simulink model "vector_model_submit_ver"  (R2023b)
settings: Solver=ode45  StartTime=0  StopTime=1  MaxStep=T_s  RelTol=1e-3  AbsTol=1e-3  EnableMultiTasking=on
values from neighbouring files (symbols this model uses):
  alpha_c = 2*pi*300    (= 1884.95559215)    [init_vector_submit_ver.m]
  alpha_s = 2*pi*20    (= 125.663706144)    [init_vector_submit_ver.m]
  J = 0.015    [init_vector_submit_ver.m]
  L_M = 0.224    [init_vector_submit_ver.m]
  L_sigma = 0.021    [init_vector_submit_ver.m]
  n_p = 2    [init_vector_submit_ver.m]
  psi_R_ref = 0.9    [init_vector_submit_ver.m]
  R_R = 2.1    [init_vector_submit_ver.m]
  T_L = 14.63    [init_vector_submit_ver.m]
  T_s = 125e-6    (= 0.000125)    [init_vector_submit_ver.m]
  tau_M_max = 20    [init_vector_submit_ver.m]
libraries: simulink x2
settings Model: Creator=mhinkkan  LastModifiedBy=Antti Jormanainen
settings SolverCC: AutoScaleAbsTol=off  AlgebraicLoopSolver=TrustRegion
settings DataIOCC: SaveFormat=Array  SignalLoggingSaveFormat=ModelDataLogs  SaveOutput=off  SignalLogging=off  DSMLogging=off  SaveTime=off  ReturnWorkspaceOutputs=off
settings OptimizationCC: BlockReduction=off  BooleanDataType=off  DefaultParameterBehavior=Inlined  OptimizeBlockIOStorage=off  BufferReuse=off  ReuseModelBlockBuffer=off  GlobalBufferReuse=off  ExpressionFolding=off  ExpressionDepthLimit=2147483647  LocalBlockOutputs=off  InitFltsAndDblsToZero=on  LifeSpan=inf
settings DebuggingCC: SaveWithParameterizedLinksMsg=none  UnderspecifiedInitializationDetection=Classic  MergeDetectMultiDrivingBlocksExec=none  SignalResolutionControl=TryResolveAllWithWarning  MultiTaskDSMMsg=warning  MultiTaskCondExecSysMsg=none  FcnCallInpInsideContextMsg=warning  UnconnectedInputMsg=warning  UnconnectedOutputMsg=warning  UnconnectedLineMsg=warning  StateNameClashWarn=warning  SFUnexpectedBacktrackingDiag=warning  SFNoUnconditionalDefaultTransitionDiag=warning  ArithmeticOperatorsInVariantConditions=warning
settings HardwareCC: ProdBitPerPointer=32  ProdBitPerSizeT=32  ProdBitPerPtrDiffT=32  ProdLargestAtomicFloat=None  ProdIntDivRoundTo=Undefined  ProdEndianess=Unspecified  ProdWordSize=32  ProdHWDeviceType=32-bit Generic  TargetUnknown=on
settings ModelReferenceCC: EnableRefExpFcnMdlSchedulingChecks=on  PropagateSignalLabelsOutOfModel=off
settings SFSimCC: SimUseLocalCustomCode=off  CustomCodeUndefinedFunction=UseInterfaceOnly
settings RTWCC: RTWUseLocalCustomCode=off
settings CodeAppCC: StateflowObjectComments=on
settings GRTTargetCC: TargetFcnLib=ansi_tfl_tmw.mat  TargetLangStandard=C89/C90 (ANSI)  CombineOutputUpdateFcns=off  GRTInterface=on
settings ConfigComp: CovMetricSettings=dw  CovSaveCumulativeToWorkspaceVar=on  CovSaveSingleToWorkspaceVar=on  CovExternalEMLEnable=off

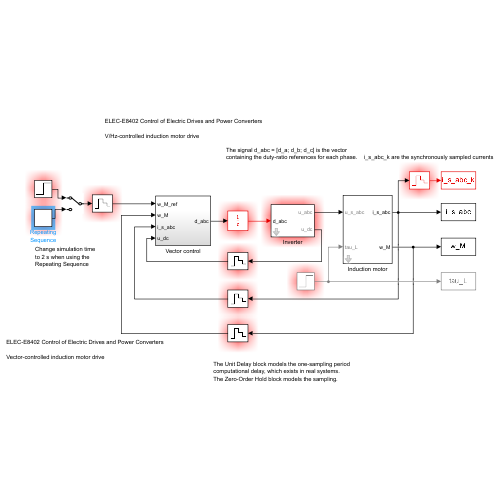
[thumbnail: Simulink's stored preview of the top-level diagram]
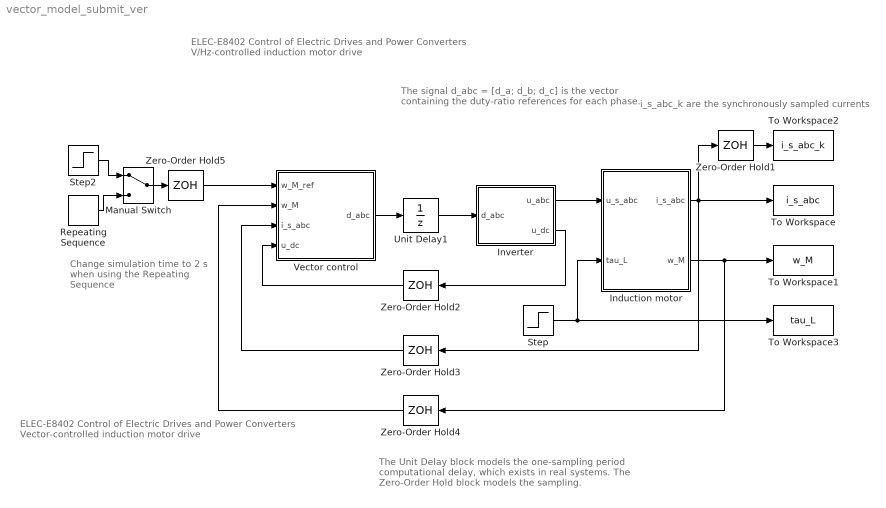
== system vector_model_submit_ver ==
  note: i_s_abc_k are the synchronously sampled currents
  note: The signal d_abc = [d_a; d_b; d_c] is the vector
      | containing the duty-ratio references for each phase.
  note: ELEC-E8402 Control of Electric Drives and Power Converters
      |
      | V/Hz-controlled induction motor drive
  note: The Unit Delay block models the one-sampling period
      | computational delay, which exists in real systems.
      | The Zero-Order Hold block models the sampling.
  note: Change simulation time
      | to 2 s when using the
      | Repeating Sequence
  note: ELEC-E8402 Control of Electric Drives and Power Converters
      |
      | Vector-controlled induction motor drive
  Induction motor : Subsystem  mask{R_s=3.7, R_R=2.1, L_sigma=0.021, L_M=0.224, n_p=2, J=0.015}
      mask prompts: R_s "Stator resistance R_s (ohm)"; R_R "Rotor resistance R_R (ohm)"; L_sigma "Leakage inductance L_sigma (H)"; L_M "Magnetizing inductance L_M (H)"; n_p "Number of pole pairs n_p"; J "Total inertia J (kgm^2)"
      mask help: Inverse-Gamma model
  Inverter : Subsystem  mask{T_s=T_s, u_dc=540}
      mask prompts: T_s "Sampling period T_s (s)"; u_dc "DC-link voltage u_dc (V)"
      mask help: The switching period is 2*Ts and the switching frequency is 1/(2*Ts).
  Manual Switch : ManualSwitch
  Repeating Sequence : simulink/Sources/Repeating Sequence  rep_seq_t=[0 .2 .8 1.2 1.8 2]  rep_seq_y=2*pi*30/n_p*[0 1 1 -1 -1 0]
  Step : Step  Time=.6  After=T_L  SampleTime=0
  Step2 : Step  Time=0.3  After=2*pi*40/n_p  SampleTime=T_s
  To Workspace : ToWorkspace  VariableName=i_s_abc  SaveFormat=Timeseries  SampleTime=-1
  To Workspace1 : ToWorkspace  VariableName=w_M  SaveFormat=Timeseries  SampleTime=-1
  To Workspace2 : ToWorkspace  VariableName=i_s_abc_k  SaveFormat=Timeseries  SampleTime=-1
  To Workspace3 : ToWorkspace  VariableName=tau_L  SaveFormat=Timeseries  SampleTime=-1
  Unit Delay1 : UnitDelay  SampleTime=T_s  HasFrameUpgradeWarning=on
  Vector control : Subsystem
  Zero-Order Hold{1..5} (5 alike) : ZeroOrderHold  SampleTime=T_s
  wires:
  Step/1 -> Induction motor/2(tau_L), To Workspace3/1
  Inverter/1(u_abc) -> Induction motor/1(u_s_abc)
  Induction motor/1(i_s_abc) -> Zero-Order Hold3/1, Zero-Order Hold1/1, To Workspace/1
  Induction motor/2(w_M) -> Zero-Order Hold4/1, To Workspace1/1
  Zero-Order Hold1/1 -> To Workspace2/1
  Manual Switch/1 -> Zero-Order Hold5/1
  Zero-Order Hold2/1 -> Vector control/4(u_dc)
  Repeating Sequence/1 -> Manual Switch/2
  Zero-Order Hold5/1 -> Vector control/1(w_M_ref)
  Step2/1 -> Manual Switch/1
  Vector control/1(d_abc) -> Unit Delay1/1
  Zero-Order Hold3/1 -> Vector control/3(i_s_abc)
  Zero-Order Hold4/1 -> Vector control/2(w_M)
  Unit Delay1/1 -> Inverter/1(d_abc)
  Inverter/2(u_dc) -> Zero-Order Hold2/1

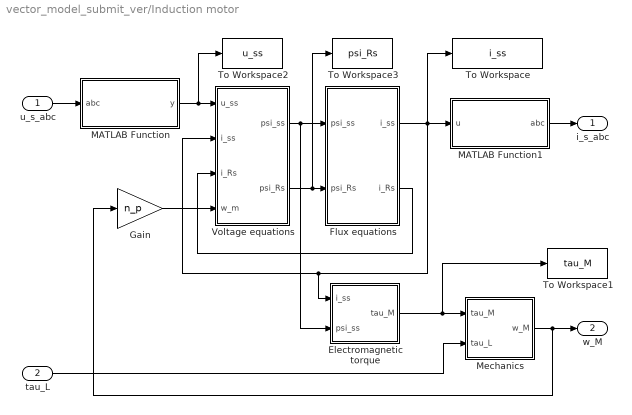
== system vector_model_submit_ver/Induction motor ==
  u_s_abc : Inport
  tau_L : Inport  Port=2
  Electromagnetic torque : Subsystem
  Flux equations : Subsystem
  Gain : Gain  Gain=n_p  SaturateOnIntegerOverflow=on  OutDataTypeStr=Inherit: Same as input  ParamDataTypeStr=Inherit: Same as input
  MATLAB Function : MATLAB Function  TreatAsAtomicUnit=on
  MATLAB Function1 : MATLAB Function  TreatAsAtomicUnit=on
  Mechanics : Subsystem
  To Workspace : ToWorkspace  VariableName=i_ss  SaveFormat=Timeseries  SampleTime=-1
  To Workspace1 : ToWorkspace  VariableName=tau_M  SaveFormat=Timeseries  SampleTime=-1
  To Workspace2 : ToWorkspace  VariableName=u_ss  SaveFormat=Timeseries  SampleTime=-1
  To Workspace3 : ToWorkspace  VariableName=psi_Rs  SaveFormat=Timeseries  SampleTime=-1
  Voltage equations : Subsystem
  i_s_abc : Outport
  w_M : Outport  Port=2
  wires:
  tau_L/1 -> Mechanics/2(tau_L)
  Mechanics/1(w_M) -> w_M/1, Gain/1
  Flux equations/1(i_ss) -> To Workspace/1, MATLAB Function1/1(u), Voltage equations/2(i_ss), Electromagnetic torque/1(i_ss)
  u_s_abc/1 -> MATLAB Function/1(abc)
  Voltage equations/2(psi_Rs) -> To Workspace3/1, Flux equations/2(psi_Rs)
  Voltage equations/1(psi_ss) -> Electromagnetic torque/2(psi_ss), Flux equations/1(psi_ss)
  Flux equations/2(i_Rs) -> Voltage equations/3(i_Rs)
  Electromagnetic torque/1(tau_M) -> To Workspace1/1, Mechanics/1(tau_M)
  MATLAB Function/1(y) -> To Workspace2/1, Voltage equations/1(u_ss)
  MATLAB Function1/1(abc) -> i_s_abc/1
  Gain/1 -> Voltage equations/4(w_m)

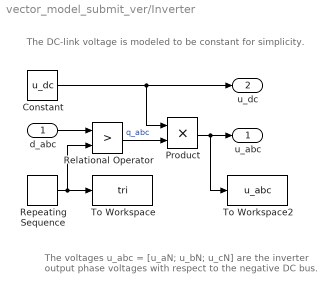
== system vector_model_submit_ver/Inverter ==
  note: The voltages u_abc = [u_aN; u_bN; u_cN] are the inverter
      | output phase voltages with respect to the negative DC bus.
  note: The DC-link voltage is modeled to be constant for simplicity.
  d_abc : Inport
  Constant : Constant  Value=u_dc  SampleTime=0
  Product : Product
  Relational Operator : RelationalOperator  Operator=>  OutDataTypeStr=boolean  InputSameDT=off
  Repeating Sequence : simulink/Sources/Repeating Sequence  rep_seq_t=[0 1 2]*T_s  rep_seq_y=[1 0 1]
  To Workspace : ToWorkspace  VariableName=tri  SaveFormat=Timeseries  SampleTime=-1
  To Workspace2 : ToWorkspace  VariableName=u_abc  SaveFormat=Timeseries  SampleTime=-1
  u_abc : Outport
  u_dc : Outport  Port=2
  wires:
  Repeating Sequence/1 -> Relational Operator/2, To Workspace/1
  d_abc/1 -> Relational Operator/1
  Relational Operator/1 -> Product/2  "q_abc"
  Constant/1 -> Product/1, u_dc/1
  Product/1 -> u_abc/1, To Workspace2/1

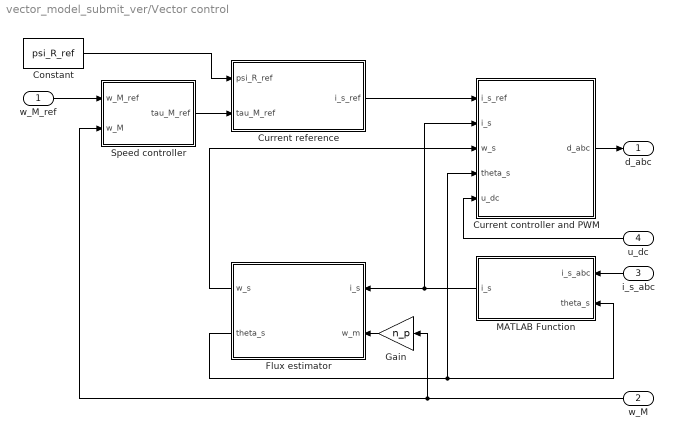
== system vector_model_submit_ver/Vector control ==
  w_M_ref : Inport
  w_M : Inport  Port=2
  i_s_abc : Inport  Port=3
  u_dc : Inport  Port=4
  Constant : Constant  Value=psi_R_ref  SampleTime=T_s
  Current controller and PWM : Subsystem
  Current reference : MATLAB Function  TreatAsAtomicUnit=on
  Flux estimator : Subsystem
  Gain : Gain  Gain=n_p  SaturateOnIntegerOverflow=on  OutDataTypeStr=Inherit: Same as input  ParamDataTypeStr=Inherit: Same as input
  MATLAB Function : MATLAB Function  TreatAsAtomicUnit=on
  Speed controller : Subsystem
  d_abc : Outport
  wires:
  Flux estimator/2(theta_s) -> Current controller and PWM/4(theta_s), MATLAB Function/2(theta_s)
  w_M/1 -> Gain/1, Speed controller/2(w_M)
  i_s_abc/1 -> MATLAB Function/1(i_s_abc)
  Current controller and PWM/1(d_abc) -> d_abc/1
  Current reference/1(i_s_ref) -> Current controller and PWM/1(i_s_ref)
  Flux estimator/1(w_s) -> Current controller and PWM/3(w_s)
  MATLAB Function/1(i_s) -> Current controller and PWM/2(i_s), Flux estimator/1(i_s)
  w_M_ref/1 -> Speed controller/1(w_M_ref)
  Constant/1 -> Current reference/1(psi_R_ref)
  u_dc/1 -> Current controller and PWM/5(u_dc)
  Speed controller/1(tau_M_ref) -> Current reference/2(tau_M_ref)
  Gain/1 -> Flux estimator/2(w_m)

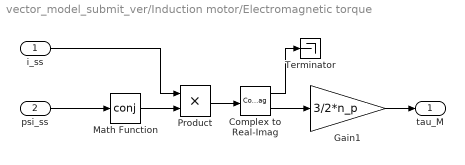
== system vector_model_submit_ver/Induction motor/Electromagnetic torque ==
  i_ss : Inport
  psi_ss : Inport  Port=2
  Complex to Real-Imag : ComplexToRealImag
  Gain1 : Gain  Gain=3/2*n_p
  Math Function : Math  Operator=conj
  Product : Product
  Terminator : Terminator
  tau_M : Outport
  wires:
  i_ss/1 -> Product/1
  Math Function/1 -> Product/2
  Product/1 -> Complex to Real-Imag/1
  Complex to Real-Imag/2 -> Gain1/1
  Gain1/1 -> tau_M/1
  psi_ss/1 -> Math Function/1
  Complex to Real-Imag/1 -> Terminator/1

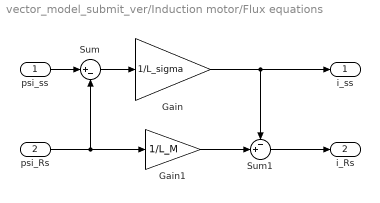
== system vector_model_submit_ver/Induction motor/Flux equations ==
  psi_ss : Inport
  psi_Rs : Inport  Port=2
  Gain : Gain  Gain=1/L_sigma
  Gain1 : Gain  Gain=1/L_M
  Sum : Sum  Inputs=|+-
  Sum1 : Sum  Inputs=-+|
  i_ss : Outport
  i_Rs : Outport  Port=2
  wires:
  psi_Rs/1 -> Gain1/1, Sum/2
  Gain1/1 -> Sum1/2
  Sum1/1 -> i_Rs/1
  psi_ss/1 -> Sum/1
  Sum/1 -> Gain/1
  Gain/1 -> Sum1/1, i_ss/1

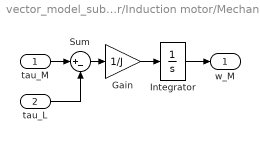
== system vector_model_submit_ver/Induction motor/Mechanics ==
  tau_M : Inport
  tau_L : Inport  Port=2
  Gain : Gain  Gain=1/J  SaturateOnIntegerOverflow=on  OutDataTypeStr=Inherit: Same as input  ParamDataTypeStr=Inherit: Same as input
  Integrator : Integrator
  Sum : Sum  Inputs=|+-  InputSameDT=on  SaturateOnIntegerOverflow=on  OutDataTypeStr=Inherit: Same as first input
  w_M : Outport
  wires:
  tau_L/1 -> Sum/2
  Sum/1 -> Gain/1
  Gain/1 -> Integrator/1
  Integrator/1 -> w_M/1
  tau_M/1 -> Sum/1

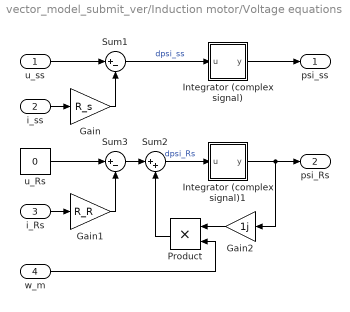
== system vector_model_submit_ver/Induction motor/Voltage equations ==
  u_ss : Inport
  i_ss : Inport  Port=2
  i_Rs : Inport  Port=3
  w_m : Inport  Port=4
  Gain : Gain  Gain=R_s
  Gain1 : Gain  Gain=R_R
  Gain2 : Gain  Gain=1j
  Integrator (complex signal) : Subsystem
      mask Display: disp('1/s');
  Integrator (complex signal)1 : Subsystem
      mask Display: disp('1/s');
  Product : Product  RndMeth=Zero
  Sum1 : Sum  Inputs=|+-
  Sum2 : Sum  Inputs=|++
  Sum3 : Sum  Inputs=|+-
  u_Rs : Constant  Value=0  SampleTime=0
  psi_ss : Outport
  psi_Rs : Outport  Port=2
  wires:
  u_ss/1 -> Sum1/1
  i_ss/1 -> Gain/1
  Sum1/1 -> Integrator (complex signal)/1(u)  "dpsi_ss"
  Gain/1 -> Sum1/2
  Integrator (complex signal)/1(y) -> psi_ss/1
  u_Rs/1 -> Sum3/1
  i_Rs/1 -> Gain1/1
  Gain1/1 -> Sum3/2
  Sum3/1 -> Sum2/1
  Sum2/1 -> Integrator (complex signal)1/1(u)  "dpsi_Rs"
  Product/1 -> Sum2/2
  Integrator (complex signal)1/1(y) -> psi_Rs/1, Gain2/1
  Gain2/1 -> Product/1
  w_m/1 -> Product/2

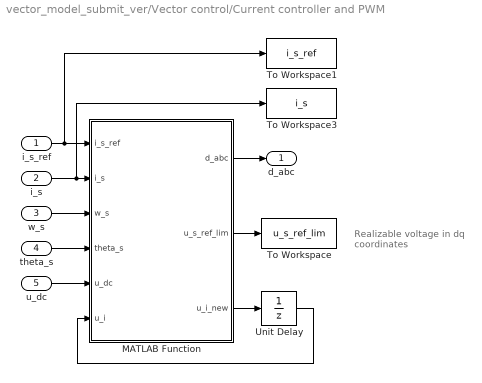
== system vector_model_submit_ver/Vector control/Current controller and PWM ==
  note: Realizable voltage
      | in dq coordinates
  i_s_ref : Inport
  i_s : Inport  Port=2
  w_s : Inport  Port=3
  theta_s : Inport  Port=4
  u_dc : Inport  Port=5
  MATLAB Function : MATLAB Function  TreatAsAtomicUnit=on
  To Workspace : ToWorkspace  VariableName=u_s_ref_lim  SaveFormat=Timeseries  SampleTime=-1
  To Workspace1 : ToWorkspace  VariableName=i_s_ref  SaveFormat=Timeseries  SampleTime=-1
  To Workspace3 : ToWorkspace  VariableName=i_s  SaveFormat=Timeseries  SampleTime=-1
  Unit Delay : UnitDelay  SampleTime=-1  HasFrameUpgradeWarning=on
  d_abc : Outport  PortDimensions=3
  wires:
  MATLAB Function/3(u_i_new) -> Unit Delay/1
  i_s_ref/1 -> To Workspace1/1, MATLAB Function/1(i_s_ref)
  w_s/1 -> MATLAB Function/3(w_s)
  i_s/1 -> To Workspace3/1, MATLAB Function/2(i_s)
  Unit Delay/1 -> MATLAB Function/6(u_i)
  theta_s/1 -> MATLAB Function/4(theta_s)
  u_dc/1 -> MATLAB Function/5(u_dc)
  MATLAB Function/1(d_abc) -> d_abc/1
  MATLAB Function/2(u_s_ref_lim) -> To Workspace/1

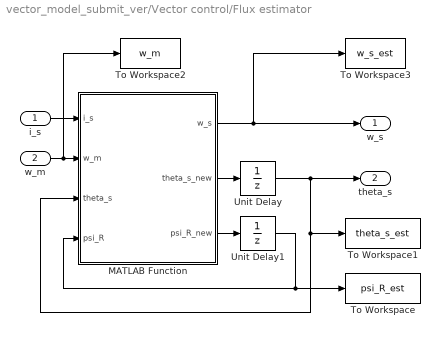
== system vector_model_submit_ver/Vector control/Flux estimator ==
  i_s : Inport
  w_m : Inport  Port=2
  MATLAB Function : MATLAB Function  TreatAsAtomicUnit=on
  To Workspace : ToWorkspace  VariableName=psi_R_est  SaveFormat=Timeseries  SampleTime=-1
  To Workspace1 : ToWorkspace  VariableName=theta_s_est  SaveFormat=Timeseries  SampleTime=-1
  To Workspace2 : ToWorkspace  VariableName=w_m  SaveFormat=Timeseries  SampleTime=-1
  To Workspace3 : ToWorkspace  VariableName=w_s_est  SaveFormat=Timeseries  SampleTime=-1
  Unit Delay : UnitDelay  SampleTime=-1  HasFrameUpgradeWarning=on
  Unit Delay1 : UnitDelay  SampleTime=-1  HasFrameUpgradeWarning=on
  w_s : Outport
  theta_s : Outport  Port=2
  wires:
  MATLAB Function/2(theta_s_new) -> Unit Delay/1
  MATLAB Function/1(w_s) -> To Workspace3/1, w_s/1
  w_m/1 -> To Workspace2/1, MATLAB Function/2(w_m)
  i_s/1 -> MATLAB Function/1(i_s)
  Unit Delay1/1 -> MATLAB Function/4(psi_R), To Workspace/1
  Unit Delay/1 -> MATLAB Function/3(theta_s), To Workspace1/1, theta_s/1
  MATLAB Function/3(psi_R_new) -> Unit Delay1/1

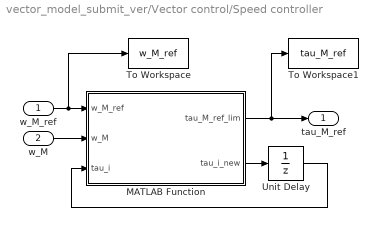
== system vector_model_submit_ver/Vector control/Speed controller ==
  w_M_ref : Inport
  w_M : Inport  Port=2
  MATLAB Function : MATLAB Function  TreatAsAtomicUnit=on
  To Workspace : ToWorkspace  VariableName=w_M_ref  SaveFormat=Timeseries  SampleTime=-1
  To Workspace1 : ToWorkspace  VariableName=tau_M_ref  SaveFormat=Timeseries  SampleTime=-1
  Unit Delay : UnitDelay  SampleTime=-1  HasFrameUpgradeWarning=on
  tau_M_ref : Outport
  wires:
  w_M_ref/1 -> To Workspace/1, MATLAB Function/1(w_M_ref)
  Unit Delay/1 -> MATLAB Function/3(tau_i)
  w_M/1 -> MATLAB Function/2(w_M)
  MATLAB Function/1(tau_M_ref_lim) -> To Workspace1/1, tau_M_ref/1
  MATLAB Function/2(tau_i_new) -> Unit Delay/1

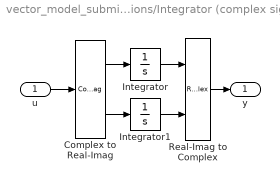
== system vector_model_submit_ver/Induction motor/Voltage equations/Integrator (complex signal) ==
  u : Inport
  Complex to Real-Imag : ComplexToRealImag
  Integrator : Integrator
  Integrator1 : Integrator
  Real-Imag to Complex : RealImagToComplex
  y : Outport
  wires:
  Complex to Real-Imag/1 -> Integrator/1
  Complex to Real-Imag/2 -> Integrator1/1
  Integrator/1 -> Real-Imag to Complex/1
  Integrator1/1 -> Real-Imag to Complex/2
  Real-Imag to Complex/1 -> y/1
  u/1 -> Complex to Real-Imag/1

== system vector_model_submit_ver/Induction motor/Voltage equations/Integrator (complex signal)1 ==
  u : Inport
  Complex to Real-Imag : ComplexToRealImag
  Integrator : Integrator
  Integrator1 : Integrator
  Real-Imag to Complex : RealImagToComplex
  y : Outport
  wires:
  Complex to Real-Imag/1 -> Integrator/1
  Complex to Real-Imag/2 -> Integrator1/1
  Integrator/1 -> Real-Imag to Complex/1
  Integrator1/1 -> Real-Imag to Complex/2
  Real-Imag to Complex/1 -> y/1
  u/1 -> Complex to Real-Imag/1

== matlab function vector_model_submit_ver/Induction motor/MATLAB Function1 ==
  data: u input size=1; abc output size=3
function abc = alphabeta2abc(u)

a = real(u);
b = real(exp(1j*4*pi/3)*u);
c = real(exp(1j*2*pi/3)*u);

abc = [a; b; c];

== matlab function vector_model_submit_ver/Induction motor/MATLAB Function ==
  data: abc input size=3; y output size=1
function y = abc2alphabeta(abc)

y = 2/3*(abc(1) + exp(1j*2*pi/3)*abc(2) + exp(1j*4*pi/3)*abc(3));

== matlab function vector_model_submit_ver/Vector control/Current controller and PWM/MATLAB Function ==
  data: i_s_ref input size=1; i_s input size=1; w_s input size=1; theta_s input size=1; u_dc input size=1; u_i input size=1; L_sigma parameter size=1; alpha_c parameter size=1; T_s parameter size=1; d_abc output size=3; u_s_ref_lim output size=1; u_i_new output
function [d_abc, u_s_ref_lim, u_i_new] = cc(i_s_ref, i_s, w_s, theta_s, ...
    u_dc, u_i, L_sigma, alpha_c, T_s)

%% Current controller 
% Gains
k_i = alpha_c^2*L_sigma;                % Integral gain
k_t = alpha_c*L_sigma;                   % Reference gain
k_p = (2*alpha_c - 1j*w_s)*L_sigma;     % Proportional gain

% Voltage reference in synchronous coordinates
u_s_ref = k_t*i_s_ref - k_p*i_s + u_i;

% Reference in stator coordinates
theta_sc = theta_s + 1.5*T_s*w_s;   % Compensation for discrete-time delays
u_ss_ref = u_s_ref*exp(1j*theta_sc);

%% Symmetrical suboscillation PWM
% Components of the voltage space vector
u_alpha_ref = real(u_ss_ref);
u_beta_ref  = imag(u_ss_ref);

% Phase-voltage references
u_a_ref = u_alpha_ref;
u_b_ref = .5*(-u_alpha_ref + sqrt(3)*u_beta_ref);
u_c_ref = .5*(-u_alpha_ref - sqrt(3)*u_beta_ref);

% Vector of phase-voltage references
u_abc_ref = [u_a_ref; u_b_ref; u_c_ref];

% Symmetrization of the references by adding the zero-sequence voltage
u0 = .5*(max(u_abc_ref) + min(u_abc_ref));
u_abc_ref = u_abc_ref - u0;

% Clamping of the reference voltages such that no phase error is caused. 
% If all phase voltage reference are realizable (below Udc/2), m = 1 holds.
m = max([2*u_abc_ref/u_dc; 1]);
u_abc_ref = u_abc_ref/m;

% Duty cycles, which can be directly used for triangle comparison, 
% if the triangle wave varies between 0...1
d_abc = .5 + u_abc_ref/u_dc;

% Realized voltage vector is calculated from the clamped duty ratios.
% If the PWM does not saturate, us_ref_lim = us_ref holds. The realized
% voltage vector is needed, e.g., for the current-controller antiwindup.
u_ss_ref_lim = 2/3*(d_abc(1) + d_abc(2)*exp(1j*2*pi/3) ...
    + d_abc(3)*exp(1j*4*pi/3))*u_dc;
% In estimated rotor flux coordinates
u_s_ref_lim = exp(-1j*theta_sc)*u_ss_ref_lim;  

%% Update the integral state of the current controller 
u_i_new = u_i + T_s*k_i*(i_s_ref - i_s + (u_s_ref_lim - u_s_ref)/k_t);

== matlab function vector_model_submit_ver/Vector control/Flux estimator/MATLAB Function ==
  data: i_s input size=1; w_m input size=1; theta_s input size=1; psi_R input size=1; R_R parameter size=1; L_M parameter size=1; T_s parameter size=1; w_s output size=1; theta_s_new output size=1; psi_R_new output size=1
function [w_s, theta_s_new, psi_R_new] = estimator(i_s, w_m, theta_s, ...
    psi_R, R_R, L_M, T_s)

% Current components
i_d = real(i_s);
i_q = imag(i_s);

% Angular frequency of the rotor flux
if(psi_R > 0) 	                    % Avoid division by zero
	w_s = w_m+R_R*i_q/psi_R;
else
	w_s = w_m;
end

% Update the states
psi_R_new = psi_R+T_s*((-R_R/L_M)*psi_R+R_R*i_d);
theta_s_new = theta_s + T_s*w_s;   	% Rotor flux angle

% Limit the angle between [-pi, pi]
while(theta_s_new > pi)
    theta_s_new = theta_s_new - 2*pi;
end
while(theta_s_new < -pi) 
    theta_s_new = theta_s_new + 2*pi;
end

== matlab function vector_model_submit_ver/Vector control/MATLAB Function ==
  data: i_s_abc input size=3; theta_s input size=1; i_s output size=1
function i_s = abc2dq(i_s_abc, theta_s)

% Phase currents
i_a = i_s_abc(1); i_b = i_s_abc(2); i_c = i_s_abc(3); 

% Space-vector transformation and coordinate transformation
i_ss = 2/3*(i_a+i_b*exp(1i*2*pi/3)+i_c*exp(1i*4*pi/3)); % abc to alfa-beeta
i_s = i_ss*exp(-1i*theta_s); 	% alfa-beeta to dq

== matlab function vector_model_submit_ver/Vector control/Current reference ==
  data: psi_R_ref input size=1; tau_M_ref input size=1; L_M parameter size=1; n_p parameter size=1; i_s_ref output size=1
function i_s_ref = curr_ref(psi_R_ref, tau_M_ref, L_M, n_p)

% Current reference in estimated rotor-flux coordinates
i_d_ref = psi_R_ref/L_M;
i_q_ref = 2*tau_M_ref/(3*n_p*psi_R_ref);

i_s_ref = i_d_ref + 1j*i_q_ref;

== matlab function vector_model_submit_ver/Vector control/Speed controller/MATLAB Function ==
  data: w_M_ref input size=1; w_M input size=1; tau_i input size=1; J parameter size=1; alpha_s parameter size=1; tau_M_max parameter size=1; tau_M_ref_lim output size=1; T_s parameter size=1; tau_i_new output
% 2DOF PI speed controller
function [tau_M_ref_lim, tau_i_new] = speed_ctrl(w_M_ref, w_M, tau_i, ...
    J, alpha_s, tau_M_max, T_s)

% Gains
k_i = alpha_s^2*J;
k_t = alpha_s*J;
k_p = 2*alpha_s*J;

% Ideal reference
tau_M_ref = k_t*w_M_ref - k_p*w_M + tau_i;

% Limited reference
tau_M_ref_lim = tau_M_ref;
if(tau_M_ref_lim > tau_M_max)
    tau_M_ref_lim = tau_M_max;
elseif(tau_M_ref_lim < -tau_M_max)
    tau_M_ref_lim = -tau_M_max;
end

% Update the integral state
tau_i_new = tau_i + T_s*k_i*(w_M_ref - w_M ...
    + (tau_M_ref_lim - tau_M_ref)/k_t);
